simulink model "Boucle_courant"  (R2016a)
settings: Solver=VariableStepAuto  StartTime=0.0  StopTime=1  RelTol=1e-3
values from neighbouring files (symbols this model uses):
  E = 24    [Script_boucle_courant.m]
  Ki = 1/Ti    (= 1000)    [Script_boucle_courant.m]
  Kp = R    (= 0.47)    [Script_boucle_courant.m]
  L = 1e-3    (= 0.001)    [Init.m]    (also in Script_boucle_courant.m = 0.00047)
  R = 1    [Init.m]    (also in Script_boucle_courant.m = 0.47)
  Te = 1/50    (= 0.02)    [Calcul_correcteur_retour_etat.m]    (also in Init.m; Script_boucle_courant.m = 0.000149253731343)
libraries: simulink x4
settings Model: Creator=dpenin  LastModifiedBy=dpenin

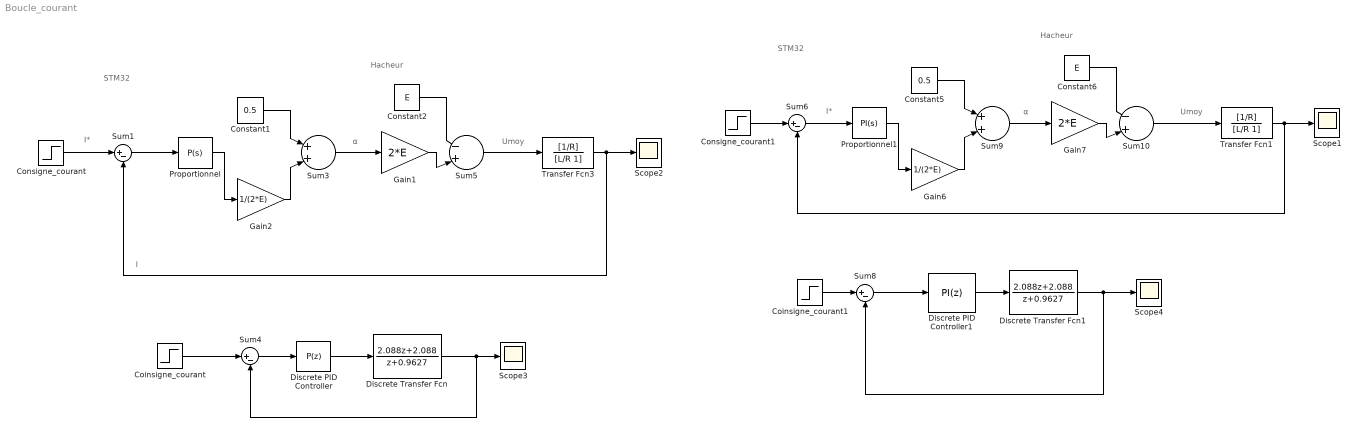
== system Boucle_courant ==
  note: Hacheur
  note: STM32
  note: I*
  note: Umoy
  note: I
  note: I*
  note: α
  note: Hacheur
  note: STM32
  note: Umoy
  note: α
  Coinsigne_courant : Step  Time=0.1  After=5  SampleTime=Te
  Coinsigne_courant1 : Step  Time=0.1  After=5  SampleTime=Te
  Consigne_courant : Step  Time=0.1  After=5  SampleTime=0
  Consigne_courant1 : Step  Time=0.1  After=5  SampleTime=0
  Constant1 : Constant  Value=0.5
  Constant2 : Constant  Value=E
  Constant5 : Constant  Value=0.5
  Constant6 : Constant  Value=E
  Discrete Transfer Fcn : DiscreteTransferFcn  Numerator=[2.088 2.088]  Denominator=[1 0.9627]  SampleTime=Te
  Discrete Transfer Fcn1 : DiscreteTransferFcn  Numerator=[2.088 2.088]  Denominator=[1 0.9627]  SampleTime=Te
  Discrete PID Controller : simulink/Continuous/PID Controller  Controller=P  TimeDomain=Discrete-time  SampleTime=Te  IntegratorMethod=Forward Euler  FilterMethod=Forward Euler  Form=Parallel  UseFilter=on  ControllerParametersSource=internal  P=Kp  I=0.001  D=0  N=100  InitialConditionSource=internal  InitialConditionForIntegrator=0.5  InitialConditionForFilter=0  ExternalReset=none  LimitOutput=on  UpperSaturationLimit=24  LowerSaturationLimit=-24  LinearizeAsGain=off  AntiWindupMode=none  Kb=1  TrackingMode=off  Kt=1  PParamMin=[]  PParamMax=[]  IParamMin=[]  IParamMax=[]  DParamMin=[]  DParamMax=[]  NParamMin=[]  NParamMax=[]  KbParamMin=[]  KbParamMax=[]  KtParamMin=[]  KtParamMax=[]  POutMin=[]  POutMax=[]  IOutMin=[]  IOutMax=[]  DOutMin=[]  DOutMax=[]  NOutMin=[]  NOutMax=[]  KbOutMin=[]  KbOutMax=[]  KtOutMin=[]  KtOutMax=[]  IntegratorOutMin=[]  IntegratorOutMax=[]  FilterOutMin=[]  FilterOutMax=[]  SumOutMin=[]  SumOutMax=[]  SumI1OutMin=[]  SumI1OutMax=[]  SumI2OutMin=[]  SumI2OutMax=[]  SumI3OutMin=[]  SumI3OutMax=[]  SumDOutMin=[]  SumDOutMax=[]  SaturationOutMin=[]  SaturationOutMax=[]  IntegratorContinuousStateAttributes=''  IntegratorStateMustResolveToSignalObject=off  IntegratorRTWStateStorageClass=Auto  FilterContinuousStateAttributes=''  FilterStateMustResolveToSignalObject=off  FilterRTWStateStorageClass=Auto  DifferentiatorICPrevScaledInput=0  DifferentiatorOutMin=[]  DifferentiatorOutMax=[]
  Discrete PID Controller1 : simulink/Continuous/PID Controller  Controller=PI  TimeDomain=Discrete-time  SampleTime=Te  IntegratorMethod=Forward Euler  FilterMethod=Forward Euler  Form=Parallel  UseFilter=on  ControllerParametersSource=internal  P=Kp  I=Ki  D=0  N=100  InitialConditionSource=internal  InitialConditionForIntegrator=0  InitialConditionForFilter=0  ExternalReset=none  LimitOutput=on  UpperSaturationLimit=24  LowerSaturationLimit=-24  LinearizeAsGain=off  AntiWindupMode=none  Kb=1  TrackingMode=off  Kt=1  PParamMin=[]  PParamMax=[]  IParamMin=[]  IParamMax=[]  DParamMin=[]  DParamMax=[]  NParamMin=[]  NParamMax=[]  KbParamMin=[]  KbParamMax=[]  KtParamMin=[]  KtParamMax=[]  POutMin=[]  POutMax=[]  IOutMin=[]  IOutMax=[]  DOutMin=[]  DOutMax=[]  NOutMin=[]  NOutMax=[]  KbOutMin=[]  KbOutMax=[]  KtOutMin=[]  KtOutMax=[]  IntegratorOutMin=[]  IntegratorOutMax=[]  FilterOutMin=[]  FilterOutMax=[]  SumOutMin=[]  SumOutMax=[]  SumI1OutMin=[]  SumI1OutMax=[]  SumI2OutMin=[]  SumI2OutMax=[]  SumI3OutMin=[]  SumI3OutMax=[]  SumDOutMin=[]  SumDOutMax=[]  SaturationOutMin=[]  SaturationOutMax=[]  IntegratorContinuousStateAttributes=''  IntegratorStateMustResolveToSignalObject=off  IntegratorRTWStateStorageClass=Auto  FilterContinuousStateAttributes=''  FilterStateMustResolveToSignalObject=off  FilterRTWStateStorageClass=Auto  DifferentiatorICPrevScaledInput=0  DifferentiatorOutMin=[]  DifferentiatorOutMax=[]
  Gain1 : Gain  Gain=2*E
  Gain2 : Gain  Gain=1/(2*E)
  Gain6 : Gain  Gain=1/(2*E)
  Gain7 : Gain  Gain=2*E
  Proportionnel : simulink/Continuous/PID Controller  Controller=P  TimeDomain=Continuous-time  SampleTime=-1  IntegratorMethod=Forward Euler  FilterMethod=Forward Euler  Form=Parallel  UseFilter=on  ControllerParametersSource=internal  P=Kp  I=7.39328094695041  D=0  N=100  InitialConditionSource=internal  InitialConditionForIntegrator=0  InitialConditionForFilter=0  ExternalReset=none  ZeroCross=off  LimitOutput=on  UpperSaturationLimit=36  LowerSaturationLimit=-36  LinearizeAsGain=on  AntiWindupMode=back-calculation  Kb=1  TrackingMode=off  Kt=1  PParamMin=[]  PParamMax=[]  IParamMin=[]  IParamMax=[]  DParamMin=[]  DParamMax=[]  NParamMin=[]  NParamMax=[]  KbParamMin=[]  KbParamMax=[]  KtParamMin=[]  KtParamMax=[]  POutMin=[]  POutMax=[]  IOutMin=[]  IOutMax=[]  DOutMin=[]  DOutMax=[]  NOutMin=[]  NOutMax=[]  KbOutMin=[]  KbOutMax=[]  KtOutMin=[]  KtOutMax=[]  IntegratorOutMin=[]  IntegratorOutMax=[]  FilterOutMin=[]  FilterOutMax=[]  SumOutMin=[]  SumOutMax=[]  SumI1OutMin=[]  SumI1OutMax=[]  SumI2OutMin=[]  SumI2OutMax=[]  SumI3OutMin=[]  SumI3OutMax=[]  SumDOutMin=[]  SumDOutMax=[]  SaturationOutMin=[]  SaturationOutMax=[]  IntegratorContinuousStateAttributes=''  IntegratorStateMustResolveToSignalObject=off  IntegratorRTWStateStorageClass=Auto  FilterContinuousStateAttributes=''  FilterStateMustResolveToSignalObject=off  FilterRTWStateStorageClass=Auto  DifferentiatorICPrevScaledInput=0  DifferentiatorOutMin=[]  DifferentiatorOutMax=[]
  Proportionnel1 : simulink/Continuous/PID Controller  Controller=PI  TimeDomain=Continuous-time  SampleTime=-1  IntegratorMethod=Forward Euler  FilterMethod=Forward Euler  Form=Parallel  UseFilter=on  ControllerParametersSource=internal  P=Kp  I=Ki  D=0  N=100  InitialConditionSource=internal  InitialConditionForIntegrator=0  InitialConditionForFilter=0  ExternalReset=none  ZeroCross=off  LimitOutput=on  UpperSaturationLimit=36  LowerSaturationLimit=-36  LinearizeAsGain=on  AntiWindupMode=back-calculation  Kb=1  TrackingMode=off  Kt=1  PParamMin=[]  PParamMax=[]  IParamMin=[]  IParamMax=[]  DParamMin=[]  DParamMax=[]  NParamMin=[]  NParamMax=[]  KbParamMin=[]  KbParamMax=[]  KtParamMin=[]  KtParamMax=[]  POutMin=[]  POutMax=[]  IOutMin=[]  IOutMax=[]  DOutMin=[]  DOutMax=[]  NOutMin=[]  NOutMax=[]  KbOutMin=[]  KbOutMax=[]  KtOutMin=[]  KtOutMax=[]  IntegratorOutMin=[]  IntegratorOutMax=[]  FilterOutMin=[]  FilterOutMax=[]  SumOutMin=[]  SumOutMax=[]  SumI1OutMin=[]  SumI1OutMax=[]  SumI2OutMin=[]  SumI2OutMax=[]  SumI3OutMin=[]  SumI3OutMax=[]  SumDOutMin=[]  SumDOutMax=[]  SaturationOutMin=[]  SaturationOutMax=[]  IntegratorContinuousStateAttributes=''  IntegratorStateMustResolveToSignalObject=off  IntegratorRTWStateStorageClass=Auto  FilterContinuousStateAttributes=''  FilterStateMustResolveToSignalObject=off  FilterRTWStateStorageClass=Auto  DifferentiatorICPrevScaledInput=0  DifferentiatorOutMin=[]  DifferentiatorOutMax=[]
  Scope{1..4} (4 alike) : Scope
  Sum{1,4,6,8} (4 alike) : Sum  Inputs=|+-
  Sum10 : Sum  Inputs=|-+|
  Sum3 : Sum  Inputs=|++|
  Sum5 : Sum  Inputs=|-+|
  Sum9 : Sum  Inputs=|++|
  Transfer Fcn1 : TransferFcn  Numerator=[1/R]  Denominator=[L/R 1]
  Transfer Fcn3 : TransferFcn  Numerator=[1/R]  Denominator=[L/R 1]
  wires:
  Coinsigne_courant/1 -> Sum4/1
  Discrete Transfer Fcn/1 -> Sum4/2, Scope3/1
  Sum4/1 -> Discrete PID Controller/1
  Coinsigne_courant1/1 -> Sum8/1
  Discrete Transfer Fcn1/1 -> Sum8/2, Scope4/1
  Sum8/1 -> Discrete PID Controller1/1
  Discrete PID Controller1/1 -> Discrete Transfer Fcn1/1
  Sum1/1 -> Proportionnel/1
  Transfer Fcn3/1 -> Sum1/2, Scope2/1
  Consigne_courant/1 -> Sum1/1
  Proportionnel/1 -> Gain2/1
  Gain2/1 -> Sum3/2
  Constant1/1 -> Sum3/1
  Sum3/1 -> Gain1/1
  Sum5/1 -> Transfer Fcn3/1
  Constant2/1 -> Sum5/1
  Gain1/1 -> Sum5/2
  Sum10/1 -> Transfer Fcn1/1
  Sum6/1 -> Proportionnel1/1
  Transfer Fcn1/1 -> Sum6/2, Scope1/1
  Proportionnel1/1 -> Gain6/1
  Gain6/1 -> Sum9/2
  Constant5/1 -> Sum9/1
  Constant6/1 -> Sum10/1
  Gain7/1 -> Sum10/2
  Sum9/1 -> Gain7/1
  Consigne_courant1/1 -> Sum6/1
  Discrete PID Controller/1 -> Discrete Transfer Fcn/1
